simulink model "Ensayo"  (R2022a)
settings: Solver=FixedStepAuto  StartTime=0.0  StopTime=inf  RelTol=1e-3
model workspace (MAT data in the model file):
  Param = Simulink.Parameter
  Param.Value = 90
  Param.DataType = 'auto'
  Param.Complexity = 'real'
  Param.Dimensions = [1 1]
  SL_ROS_VariableLengthArrays_MaxSizes.CommonInfo.ArrayTruncateAction = 'EmitWarning'
  SL_ROS_VariableLengthArrays_MaxSizes.MsgTypeMap = containers.Map
  SL_ROS_VariableLengthArrays_MaxSizes.MsgTypeMap.serialization.keys = {'sensor_msgs/LaserScan'}
  SL_ROS_VariableLengthArrays_MaxSizes.MsgTypeMap.serialization.values{1}(1).PropertyName = 'intensities'
  SL_ROS_VariableLengthArrays_MaxSizes.MsgTypeMap.serialization.values{1}(1).DataType = 'single'
  SL_ROS_VariableLengthArrays_MaxSizes.MsgTypeMap.serialization.values{1}(1).MaxLength = 360
  SL_ROS_VariableLengthArrays_MaxSizes.MsgTypeMap.serialization.values{1}(2).PropertyName = 'ranges'
  SL_ROS_VariableLengthArrays_MaxSizes.MsgTypeMap.serialization.values{1}(2).DataType = 'single'
  SL_ROS_VariableLengthArrays_MaxSizes.MsgTypeMap.serialization.values{1}(2).MaxLength = 360
  SL_ROS_VariableLengthArrays_MaxSizes.MsgTypeMap.serialization.uniformity = 0
  SL_ROS_VariableLengthArrays_MaxSizes.MsgTypeMap.serialization.keyType = 'char'
  SL_ROS_VariableLengthArrays_MaxSizes.MsgTypeMap.serialization.valueType = 'any'
undefined symbols (not defined in the file): angular, header, linear, temperature
libraries: ros2lib x6, dspstat3 x2, simulink_extras x1
settings Model: Creator=Francisco  LastModifiedBy=Francisco
settings OptimizationCC: EnhancedBackFolding=on  PassReuseOutputArgsAs=Individual arguments  ZeroExternalMemoryAtStartup=off  ZeroInternalMemoryAtStartup=off  MaxStackSize=64  OptimizeBlockOrder=speed  DifferentSizesBufferReuse=on  OptimizationCustomize=off  EfficientTunableParamExpr=on
settings DebuggingCC: ParameterTunabilityLossMsg=error
settings SFSimCC: MATLABDynamicMemAlloc=off
settings RTWCC: SystemTargetFile=ert.tlc  HardwareBoard=Robot Operating System 2 (ROS 2)  TLCOptions="-aInlineSetEventsForThisBaseRateFcn=TLC_FALSE -aSuppressMultiTaskScheduler=TLC_FALSE  -aRateBasedStepFcn=0"  TemplateMakefile=ert_default_tmf  Toolchain=Colcon Tools  TargetLang=C++
settings CodeAppCC: ForceParamTrailComments=on  IgnoreCustomStorageClasses=off  OperatorAnnotations=on  SimulinkDataObjDesc=on  SFDataObjDesc=on  InsertBlockDesc=on
settings ERTTargetCC: CodeInterfacePackaging=C++ class  SupportContinuousTime=on  RootIOFormat=Structure reference

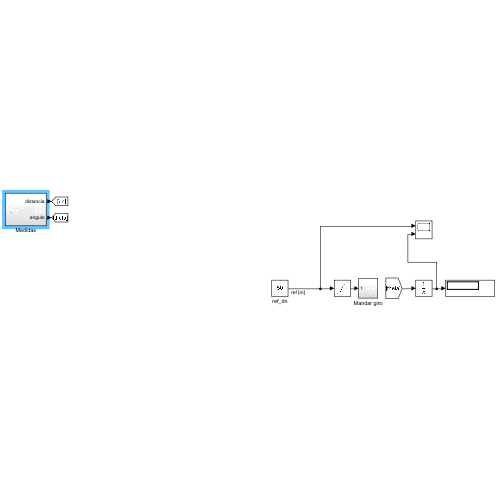
[thumbnail: Simulink's stored preview of the top-level diagram]
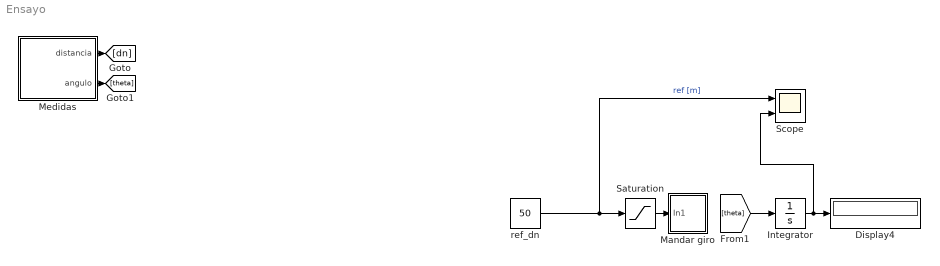
== system Ensayo ==
  Display4 : Display
  Integrator : Integrator
  Mandar giro : Subsystem
  Medidas : Subsystem
  Saturation : Saturate  UpperLimit=100  LowerLimit=-100  LinearizeAsGain=off
  Scope : Scope  NumInputPorts=2
  ref_dn : Constant  Value=50
  wires:
  Saturation/1 -> Mandar giro/1(In1)
  Medidas/1(distancia) -> [dn]
  Medidas/2(angulo) -> [theta]
  [theta] -> Integrator/1
  Integrator/1 -> Scope/2, Display4/1
  ref_dn/1 -> Scope/1, Saturation/1  "ref [m]"

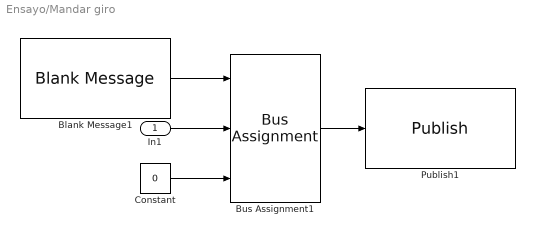
== system Ensayo/Mandar giro ==
  In1 : Inport
  Blank Message1 : ros2lib/Blank Message  messageClass=Message  entityType=geometry_msgs/Twist  messageType=geometry_msgs/Twist  SampleTime=inf
      settings: SourceProductBaseCode=RR
  Bus Assignment1 : BusAssignment  AssignedSignals=angular.z,linear.x
  Constant : Constant  Value=0
  Publish1 : ros2lib/Publish  topicSource=Select from ROS network  topic=/cmd_vel  messageType=geometry_msgs/Twist  QOSHistory=Keep last  QOSDepth=1  QOSReliability=Reliable  QOSDurability=Volatile
      settings: SourceProductBaseCode=RR
  wires:
  Bus Assignment1/1 -> Publish1/1
  Blank Message1/1 -> Bus Assignment1/1
  In1/1 -> Bus Assignment1/2
  Constant/1 -> Bus Assignment1/3

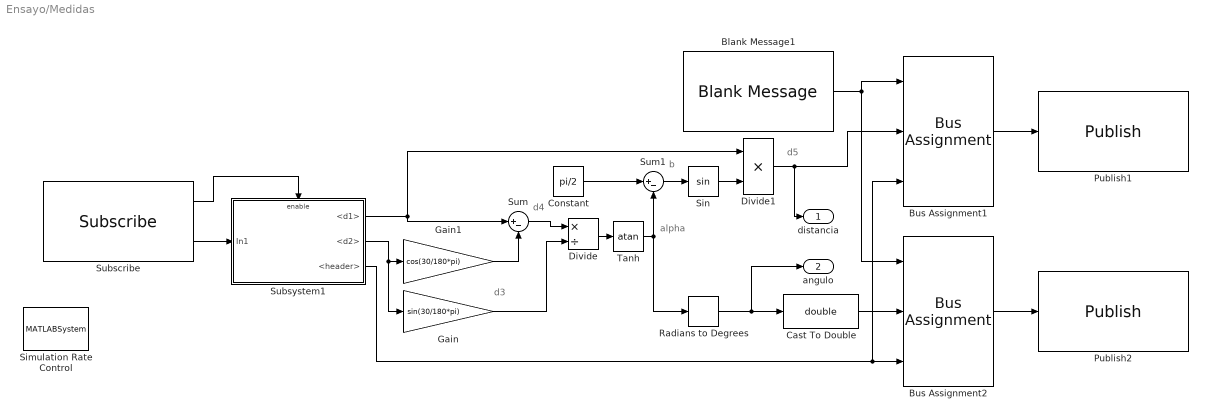
== system Ensayo/Medidas ==
  note: d5
  note: b
  note: alpha
  note: d3
  note: d4
  Blank Message1 : ros2lib/Blank Message  messageClass=Message  entityType=sensor_msgs/Temperature  messageType=sensor_msgs/Temperature  SampleTime=1/360
      settings: SourceProductBaseCode=RR
  Bus Assignment1 : BusAssignment  AssignedSignals=temperature,header
  Bus Assignment2 : BusAssignment  AssignedSignals=temperature,header
  Cast To Double : DataTypeConversion  OutDataTypeStr=double  SaturateOnIntegerOverflow=off  RndMeth=Floor
  Constant : Constant  Value=pi/2
  Divide : Product  Inputs=*/
  Divide1 : Product  Inputs=**
  Gain : Gain  Gain=sin(30/180*pi)
  Gain1 : Gain  Gain=cos(30/180*pi)
  Publish1 : ros2lib/Publish  topicSource=Specify your own  topic=/distanciaPared  messageType=sensor_msgs/Temperature  QOSHistory=Keep last  QOSDepth=1  QOSReliability=Reliable  QOSDurability=Volatile
      settings: SourceProductBaseCode=RR
  Publish2 : ros2lib/Publish  topicSource=Specify your own  topic=/anguloPared  messageType=sensor_msgs/Temperature  QOSHistory=Keep last  QOSDepth=1  QOSReliability=Reliable  QOSDurability=Volatile
      settings: SourceProductBaseCode=RR
  Radians to Degrees : simulink_extras/Transformations/Radians to Degrees
  Simulation Rate Control : MATLABSystem  System=ExampleHelperSimulationRateControl  SampleTime=0.01
      mask Type: ExampleHelperSimulationRateControl
      mask Display: disp('Rate Control');
  Sin : Trigonometry
  Subscribe : ros2lib/Subscribe  topicSource=Select from ROS network  topic=/scan  messageType=sensor_msgs/LaserScan  sampleTime=-1  QOSHistory=Keep last  QOSDepth=10  QOSReliability=Best effort  QOSDurability=Volatile
      settings: SourceProductBaseCode=RR
  Subsystem1 : Subsystem
  Sum : Sum  Inputs=|+-
  Sum1 : Sum  Inputs=|+-
  Tanh : Trigonometry  Operator=atan
  distancia : Outport
  angulo : Outport  Port=2
  wires:
  Subscribe/1 -> Subsystem1/Enable
  Constant/1 -> Sum1/1
  Subsystem1/1(<d1>) -> Sum/1, Divide1/1
  Subsystem1/2(<d2>) -> Gain/1, Gain1/1
  Subscribe/2 -> Subsystem1/1(In1)
  Cast To Double/1 -> Bus Assignment2/2
  Gain/1 -> Divide/2
  Sum/1 -> Divide/1
  Gain1/1 -> Sum/2
  Sin/1 -> Divide1/2
  Tanh/1 -> Sum1/2, Radians to Degrees/1
  Divide/1 -> Tanh/1
  Radians to Degrees/1 -> angulo/1, Cast To Double/1
  Subsystem1/3(<header>) -> Bus Assignment1/3, Bus Assignment2/3
  Sum1/1 -> Sin/1
  Bus Assignment1/1 -> Publish1/1
  Bus Assignment2/1 -> Publish2/1
  Blank Message1/1 -> Bus Assignment2/1, Bus Assignment1/1
  Divide1/1 -> distancia/1, Bus Assignment1/2

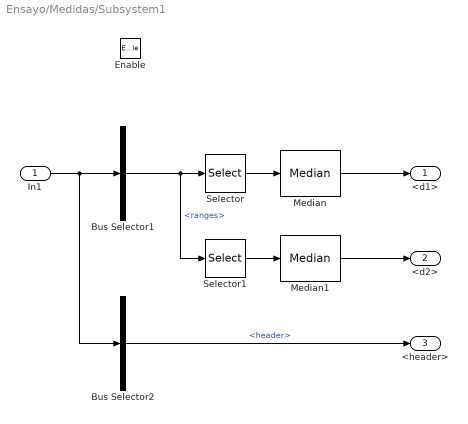
== system Ensayo/Medidas/Subsystem1 ==
  In1 : Inport
  Enable : EnablePort
  Bus Selector1 : BusSelector  OutputSignals=ranges
  Bus Selector2 : BusSelector  OutputSignals=header
  Median : dspstat3/Median  sortAlg=Quick sort  directionMode=Each column  dimension=1  roundingMode=Floor  overflowMode=off  accumDataTypeStr=Inherit: Same as product output  accumLastDataTypeStr=Inherit: Same as product output  outputDataTypeStr=Inherit: Same as accumulator  outputMin=[]  outputMax=[]  outputLastDataTypeStr=Inherit: Same as accumulator
      settings: SourceProductBaseCode=DS  allowOverrides=off
  Median1 : dspstat3/Median  sortAlg=Quick sort  directionMode=Each column  dimension=1  roundingMode=Floor  overflowMode=off  accumDataTypeStr=Inherit: Same as product output  accumLastDataTypeStr=Inherit: Same as product output  outputDataTypeStr=Inherit: Same as accumulator  outputMin=[]  outputMax=[]  outputLastDataTypeStr=Inherit: Same as accumulator
      settings: SourceProductBaseCode=DS  allowOverrides=off
  Selector : Selector  IndexMode=Zero-based  InputPortWidth=360  IndexOptions=Index vector (dialog)  Indices=[88:92]  OutputSizes=1
  Selector1 : Selector  IndexMode=Zero-based  InputPortWidth=360  IndexOptions=Index vector (dialog)  Indices=[118:122]  OutputSizes=1
  <d1> : Outport
  <d2> : Outport  Port=2
  <header> : Outport  Port=3
  wires:
  In1/1 -> Bus Selector2/1, Bus Selector1/1
  Bus Selector1/1 -> Selector1/1, Selector/1  "<ranges>"
  Selector/1 -> Median/1
  Selector1/1 -> Median1/1
  Median/1 -> <d1>/1
  Median1/1 -> <d2>/1
  Bus Selector2/1 -> <header>/1  "<header>"
